simulink model "pendulum"  (R2025b)
settings: Solver=VariableStepAuto  StartTime=0.0  StopTime=50  RelTol=1e-3
values from neighbouring files (symbols this model uses):
  b = 0.5    [untitled.m]
  g = 9.81    [untitled.m]
undefined symbols (not defined in the file or in its folder): pendulum_func
settings Model: Creator=la  LastModifiedBy=seby
settings SolverCC: AlgebraicLoopSolver=TrustRegion
settings DataIOCC: Refine=10
settings DebuggingCC: UnconnectedInputMsg=warning  UnconnectedOutputMsg=warning  UnconnectedLineMsg=warning
settings ModelReferenceCC: EnableRefExpFcnMdlSchedulingChecks=on
settings RTWCC: GPUComputeCapability=3.5

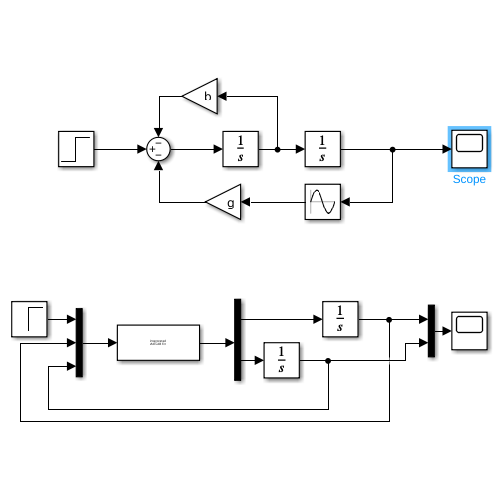
[thumbnail: Simulink's stored preview of the top-level diagram]
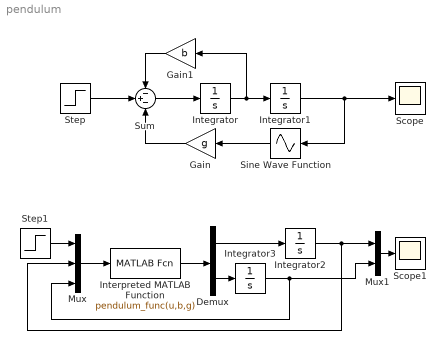
== system pendulum ==
  Demux : Demux  Outputs=2
  Gain : Gain  Gain=g
  Gain1 : Gain  Gain=b
  Integrator{,1..3} (4 alike) : Integrator
  Interpreted MATLAB Function : MATLABFcn  MATLABFcn=pendulum_func(u,b,g)
  Mux : Mux  Inputs=3
  Mux1 : Mux  Inputs=2
  Scope : Scope
      settings: ActiveDisplayYMinimum=-0.022708152280968324  ActiveDisplayYMaximum=0.20437337052871496
  Scope1 : Scope
      settings: ActiveDisplayYMinimum=-1  ActiveDisplayYMaximum=1
  Sine Wave Function : Sin  TimeSource=Use external signal  SampleTime=0
  Step : Step  SampleTime=0
  Step1 : Step  SampleTime=0
  Sum : Sum  Inputs=-+-
  wires:
  Step/1 -> Sum/2
  Sine Wave Function/1 -> Gain/1
  Sum/1 -> Integrator/1
  Integrator/1 -> Gain1/1, Integrator1/1
  Integrator1/1 -> Scope/1, Sine Wave Function/1
  Gain/1 -> Sum/3
  Gain1/1 -> Sum/1
  Mux/1 -> Interpreted MATLAB Function/1
  Step1/1 -> Mux/1
  Interpreted MATLAB Function/1 -> Demux/1
  Demux/1 -> Integrator2/1
  Demux/2 -> Integrator3/1
  Integrator2/1 -> Mux/2, Mux1/1
  Integrator3/1 -> Mux1/2, Mux/3
  Mux1/1 -> Scope1/1
